simulink library "lib_accessory2"  (Simulink 4.1.1)
values from neighbouring files (symbols this model uses):
  logFlag = 1    [advSACompMaskInit.m]    (also in advSACompMaskInitR13.m)
undefined symbols (not defined in the file or in its folder): acc_abc_dutycycle, acc_abc_init, acc_ac_dutycycle, acc_ac_init, acc_acdc_inverter_eff, acc_alt_init, acc_dcdc_eff, acc_ef_dutycycle, acc_ef_init, acc_elec_eff, acc_elec_efficiency, acc_elec_pwr, acc_mech_eff, acc_mech_pwr, acc_mech_trq, acc_op_dutycycle, acc_op_init, acc_ps_dutycycle, acc_ps_init, acc_sindafile, acc_wp_dutycycle, acc_wp_init, amb_tmp, ess_on, fc_on, generalName, map_spd, max_pwr, tc_gc_to_fc_ratio, time_step, vc_idle_bool, vc_idle_spd, vinf
libraries: lib_cosimulation x29, lib_accessory2 x15, lib_outputs x11, simulink3 x10, lib_accessory x8, lib_etc x2
(part 4 of 5)

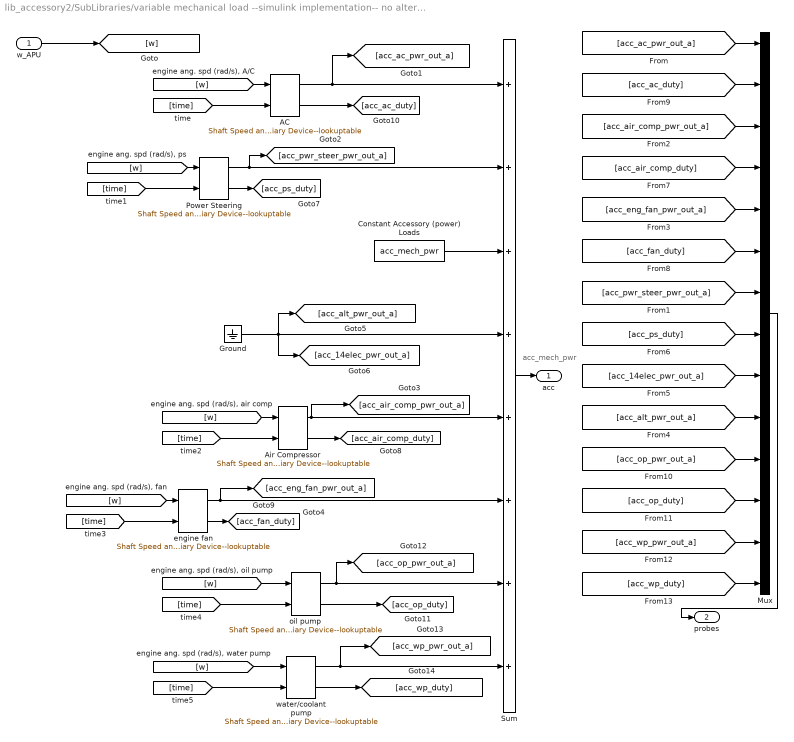
== system lib_accessory2/SubLibraries/variable mechanical load --simulink implementation-- no alternator ==
  note: acc_mech_pwr
  w_APU : Inport  Port=1  LatchInput=off
  AC : lib_accessory/SubLibraries/Shaft Speed and Time Loaded Auxiliary Device--lookuptable  fname=acc_ac_init  acc_duty=acc_ac_dutycycle
  Air Compressor : lib_accessory/SubLibraries/Shaft Speed and Time Loaded Auxiliary Device--lookuptable  fname=acc_abc_init  acc_duty=acc_abc_dutycycle
  Constant Accessory (power) Loads : Constant  Value=acc_mech_pwr
  Ground : Ground
  Mux : Mux  Inputs=14
  Power Steering : lib_accessory/SubLibraries/Shaft Speed and Time Loaded Auxiliary Device--lookuptable  fname=acc_ps_init  acc_duty=acc_ps_dutycycle
  Sum : Sum  Inputs=++++++++  SaturateOnIntegerOverflow=on
  engine fan : lib_accessory/SubLibraries/Shaft Speed and Time Loaded Auxiliary Device--lookuptable  fname=acc_ef_init  acc_duty=acc_ef_dutycycle
  oil pump : lib_accessory/SubLibraries/Shaft Speed and Time Loaded Auxiliary Device--lookuptable  fname=acc_op_init  acc_duty=acc_op_dutycycle
  water/coolant pump : lib_accessory/SubLibraries/Shaft Speed and Time Loaded Auxiliary Device--lookuptable  fname=acc_wp_init  acc_duty=acc_wp_dutycycle
  acc : Outport  Port=1
  probes : Outport  Port=2
  wires:
  [time] -> AC/2
  [w] -> AC/1
  AC/2 -> [acc_ac_duty]
  AC/1 -> Sum/1, [acc_ac_pwr_out_a]
  Constant Accessory (power) Loads/1 -> Sum/3
  Sum/1 -> acc/1
  Air Compressor/2 -> [acc_air_comp_duty]
  Air Compressor/1 -> Sum/5, [acc_air_comp_pwr_out_a]
  [w] -> Air Compressor/1
  [time] -> Air Compressor/2
  oil pump/1 -> [acc_op_pwr_out_a], Sum/7
  oil pump/2 -> [acc_op_duty]
  [time] -> oil pump/2
  [w] -> oil pump/1
  engine fan/2 -> [acc_fan_duty]
  [time] -> engine fan/2
  engine fan/1 -> Sum/6, [acc_eng_fan_pwr_out_a]
  [w] -> engine fan/1
  Power Steering/2 -> [acc_ps_duty]
  [w] -> Power Steering/1
  [time] -> Power Steering/2
  Power Steering/1 -> Sum/2, [acc_pwr_steer_pwr_out_a]
  w_APU/1 -> [w]
  [acc_ac_pwr_out_a] -> Mux/1
  Ground/1 -> Sum/4, [acc_alt_pwr_out_a], [acc_14elec_pwr_out_a]
  Mux/1 -> probes/1
  water/coolant pump/1 -> Sum/8, [acc_wp_pwr_out_a]
  [time] -> water/coolant pump/2
  [w] -> water/coolant pump/1
  water/coolant pump/2 -> [acc_wp_duty]
  [acc_ac_duty] -> Mux/2
  [acc_air_comp_pwr_out_a] -> Mux/3
  [acc_air_comp_duty] -> Mux/4
  [acc_eng_fan_pwr_out_a] -> Mux/5
  [acc_fan_duty] -> Mux/6
  [acc_pwr_steer_pwr_out_a] -> Mux/7
  [acc_ps_duty] -> Mux/8
  [acc_14elec_pwr_out_a] -> Mux/9
  [acc_alt_pwr_out_a] -> Mux/10
  [acc_op_pwr_out_a] -> Mux/11
  [acc_op_duty] -> Mux/12
  [acc_wp_pwr_out_a] -> Mux/13
  [acc_wp_duty] -> Mux/14

== system lib_accessory2/ACC ELEC <acce>/ACC ELEC model and interface/electrical accessory model ==
  note: Backward-Forward Models
  "requested electrical Power, out to the driveline (W)" : Inport  Port=1  LatchInput=off
  achieved power in from power source (W) : Inport  Port=2  LatchInput=off
  Block NOTES : Subsystem
      settings: RTWFcnNameOpts=Auto  RTWFileNameOpts=Auto
      mask Display: disp('Block\nNOTES')
  backward model : Subsystem
      settings: RTWFcnNameOpts=Auto  RTWFileNameOpts=Auto
  electrical power logging : lib_accessory2/SubLibraries/electrical power logging  eff=acc_mech_eff
      link override enhancedToWorkspace1/To Workspace: VariableName=acce_elec_pwr_in_a  SampleTime=-1  SaveFormat=Array
  enhancedToWorkspace : Subsystem  TreatAsAtomicUnit=on  mask(enhancedToWorkspace){generalName=generalName, specificName=elec_pwr_a, logFlag=logFlag}
      mask prompts: generalName "General Name [char-evaluated]"; specificName "Specific Name [char-literal]"; logFlag "Enable flag (1=on,0=off)"
      mask help: A wrapper for the Simulink "To Workspace" block that allows you to evaluate the name of the variable to log to workspace. This is useful to avoid the double logging errors that occur when you pull in two library models that attempt to log to the same variable.
      mask init:
      | enhancedToWsMaker
      settings: CopyFcn=breakLinkCopyFcn  ParentCloseFcn=breakLinkParCloseFcn  RTWFcnNameOpts=Auto  RTWFileNameOpts=Auto
      mask Help:
      | <h2>Enhanced To Workspace Block</h2>
      | <h3>Parameters</h3>
      | <UL>
      | <li><b>General Name:</b> This is the more general name of the variable. Variables are saved to the workspace as <i>generalName_specificName</i>. Note that this is an evaluated variable. If you would like to type in the value directly, it must be surrounded with single quotes. Otherwise you can input the name of a variable containing a char string.</li>
      | <li><b>Specific Name:</b> This is the specific name of the variable. Note that this is input as a char literal (i.e., you don't need quotes).</li>
      | <li><b>Enable Flag:</b> This flag should have the value of 0 or 1. If 0, the variable will not be logged to the workspace. If 1, the variable will be logged. This is done so that variable logging can be turned off to improve speed.</li>
      | </ul>
      | <h3>Overview</h3>
      | <p>The enhanced to workspace block was put together to allow one to dynamically resolve variable names at run time in simulink. This is most powerful when used in conjunction with a masked subsystem to allow multiple instances of that masked subsytem to be used in the same model. The strategy is to set the generalName in the block mask which will allow the block to change the general name for all variable logging on the fly.
      | <h3>Helper Files</h3>
      | <p>Three m-files are required by the enhancedToWorkspace block. These files are located in the &lt; ADVISOR root &gt;/GUI directory :
      | <ul>
      | <li><i>enhancedToWsMaker.m</i> This file runs the mask initialization for the block</li>
      | <li><i>breakLinkCopyFcn.m</i> This file is used by the block callback when the simulink block is copied. It is necessary to break the link to the enhancedToWorkspace similar to the To Workspace block in order for it to be able to configure itself. (Try copying simulink's To Workspace block--it is impossible to make a link)</li>
      | <li><i>breakLinkParCloseFcn.m</i> This file is similar to the breakLinkCopyFcn and is used when a parent system is closed</li>
      | </ul>
      | <hr>
      | 
      | <p>Created 2003-Jan-21, Michael Patrick O'Keefe, NREL</p>
      | 
      | <!--
      | <VARDEF>
      | <H3>var_name</H3>
      | <UL>
      | <LI><B>data type</B> data type here</LI>
      | <LI><B>units</B> units here</LI>
      | <LI><B>vehicle type</B> vehicle type here</LI>
      | <LI><B>description</B> description here</LI>
      | </UL>
      | </VARDEF>
      | -->
      mask Display: disp([generalName,'_',specificName])
  enhancedToWorkspace1 : Subsystem  TreatAsAtomicUnit=on  mask(enhancedToWorkspace){generalName=generalName, specificName=elec_pwr_r, logFlag=logFlag}
      mask prompts: generalName "General Name [char-evaluated]"; specificName "Specific Name [char-literal]"; logFlag "Enable flag (1=on,0=off)"
      mask help: A wrapper for the Simulink "To Workspace" block that allows you to evaluate the name of the variable to log to workspace. This is useful to avoid the double logging errors that occur when you pull in two library models that attempt to log to the same variable.
      mask init:
      | enhancedToWsMaker
      settings: CopyFcn=breakLinkCopyFcn  ParentCloseFcn=breakLinkParCloseFcn  RTWFcnNameOpts=Auto  RTWFileNameOpts=Auto
      mask Help:
      | <h2>Enhanced To Workspace Block</h2>
      | <h3>Parameters</h3>
      | <UL>
      | <li><b>General Name:</b> This is the more general name of the variable. Variables are saved to the workspace as <i>generalName_specificName</i>. Note that this is an evaluated variable. If you would like to type in the value directly, it must be surrounded with single quotes. Otherwise you can input the name of a variable containing a char string.</li>
      | <li><b>Specific Name:</b> This is the specific name of the variable. Note that this is input as a char literal (i.e., you don't need quotes).</li>
      | <li><b>Enable Flag:</b> This flag should have the value of 0 or 1. If 0, the variable will not be logged to the workspace. If 1, the variable will be logged. This is done so that variable logging can be turned off to improve speed.</li>
      | </ul>
      | <h3>Overview</h3>
      | <p>The enhanced to workspace block was put together to allow one to dynamically resolve variable names at run time in simulink. This is most powerful when used in conjunction with a masked subsystem to allow multiple instances of that masked subsytem to be used in the same model. The strategy is to set the generalName in the block mask which will allow the block to change the general name for all variable logging on the fly.
      | <h3>Helper Files</h3>
      | <p>Three m-files are required by the enhancedToWorkspace block. These files are located in the &lt; ADVISOR root &gt;/GUI directory :
      | <ul>
      | <li><i>enhancedToWsMaker.m</i> This file runs the mask initialization for the block</li>
      | <li><i>breakLinkCopyFcn.m</i> This file is used by the block callback when the simulink block is copied. It is necessary to break the link to the enhancedToWorkspace similar to the To Workspace block in order for it to be able to configure itself. (Try copying simulink's To Workspace block--it is impossible to make a link)</li>
      | <li><i>breakLinkParCloseFcn.m</i> This file is similar to the breakLinkCopyFcn and is used when a parent system is closed</li>
      | </ul>
      | <hr>
      | 
      | <p>Created 2003-Jan-21, Michael Patrick O'Keefe, NREL</p>
      | 
      | <!--
      | <VARDEF>
      | <H3>var_name</H3>
      | <UL>
      | <LI><B>data type</B> data type here</LI>
      | <LI><B>units</B> units here</LI>
      | <LI><B>vehicle type</B> vehicle type here</LI>
      | <LI><B>description</B> description here</LI>
      | </UL>
      | </VARDEF>
      | -->
      mask Display: disp([generalName,'_',specificName])
  forward model : Subsystem
      settings: RTWFcnNameOpts=Auto  RTWFileNameOpts=Auto
  "requested electrical Power, in from the power source (W)" : Outport  Port=1
  "achieved electrical Power, out to the driveline (W)" : Outport  Port=2
  tag scope: acc_elec_pwr_a=scoped, acc_elec_pwr_r=scoped
  wires:
  "requested electrical Power, out to the driveline (W)"/1 -> backward model/1(pwr_in)
  backward model/1(elec_out) -> "requested electrical Power, in from the power source (W)"/1
  achieved power in from power source (W)/1 -> forward model/1(pwr_in)
  forward model/1(pwr_out) -> "achieved electrical Power, out to the driveline (W)"/1
  backward model/2(elec_acc_out) -> [acc_elec_pwr_r], forward model/2(acc_pwr_in), enhancedToWorkspace1/1(In1)
  forward model/2(acc_pwr_out) -> [acc_elec_pwr_a], enhancedToWorkspace/1(In1), electrical power logging/1

== system lib_accessory2/ACC ELEC <acce>/ACC ELEC model and interface/signal annotator ==
  In1 : Inport  Port=1  LatchInput=off
  Out1 : Outport  Port=1
  wires:
  In1/1 -> Out1/1  "driveline_elec_pwr_r"

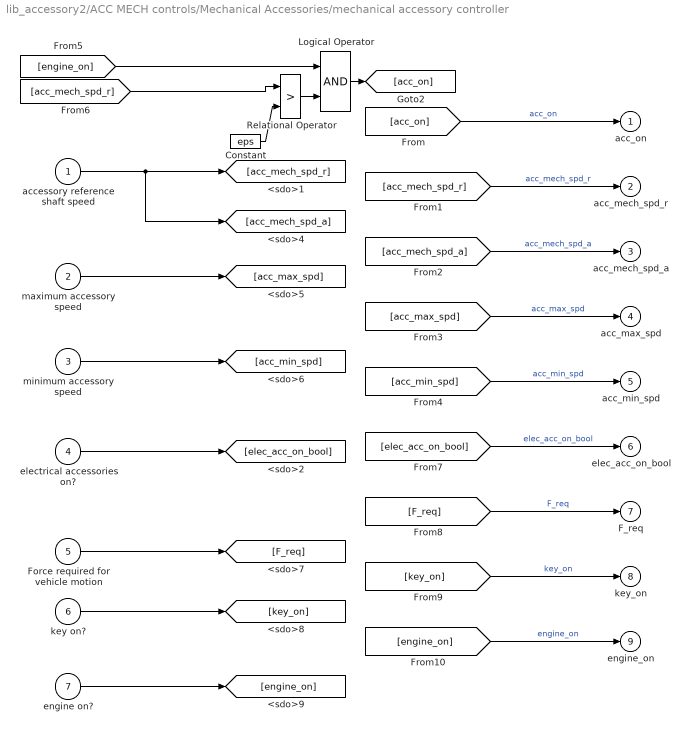
== system lib_accessory2/ACC MECH controls/Mechanical Accessories/mechanical accessory controller ==
  accessory reference shaft speed : Inport  Port=1  LatchInput=off
  maximum accessory speed : Inport  Port=2  LatchInput=off
  minimum accessory speed : Inport  Port=3  LatchInput=off
  electrical accessories on? : Inport  Port=4  LatchInput=off
  Force required for vehicle motion : Inport  Port=5  LatchInput=off
  key on? : Inport  Port=6  LatchInput=off
  engine on? : Inport  Port=7  LatchInput=off
  Constant : Constant  Value=eps
  Logical Operator : Logic  Operator=AND  Inputs=2
  Relational Operator : RelationalOperator  Operator=>
  acc_on : Outport  Port=1  InitialOutput=0
  acc_mech_spd_r : Outport  Port=2  InitialOutput=0
  acc_mech_spd_a : Outport  Port=3  InitialOutput=0
  acc_max_spd : Outport  Port=4  InitialOutput=0
  acc_min_spd : Outport  Port=5  InitialOutput=0
  elec_acc_on_bool : Outport  Port=6  InitialOutput=0
  F_req : Outport  Port=7  InitialOutput=0
  key_on : Outport  Port=8  InitialOutput=0
  engine_on : Outport  Port=9  InitialOutput=0
  wires:
  accessory reference shaft speed/1 -> [acc_mech_spd_r], [acc_mech_spd_a]
  maximum accessory speed/1 -> [acc_max_spd]
  minimum accessory speed/1 -> [acc_min_spd]
  electrical accessories on?/1 -> [elec_acc_on_bool]
  Force required for vehicle motion/1 -> [F_req]
  key on?/1 -> [key_on]
  engine on?/1 -> [engine_on]
  [acc_mech_spd_r] -> Relational Operator/1
  Constant/1 -> Relational Operator/2
  [engine_on] -> Logical Operator/1
  Relational Operator/1 -> Logical Operator/2
  Logical Operator/1 -> [acc_on]
  [acc_on] -> acc_on/1  "acc_on"
  [engine_on] -> engine_on/1  "engine_on"
  [key_on] -> key_on/1  "key_on"
  [F_req] -> F_req/1  "F_req"
  [elec_acc_on_bool] -> elec_acc_on_bool/1  "elec_acc_on_bool"
  [acc_min_spd] -> acc_min_spd/1  "acc_min_spd"
  [acc_max_spd] -> acc_max_spd/1  "acc_max_spd"
  [acc_mech_spd_a] -> acc_mech_spd_a/1  "acc_mech_spd_a"
  [acc_mech_spd_r] -> acc_mech_spd_r/1  "acc_mech_spd_r"

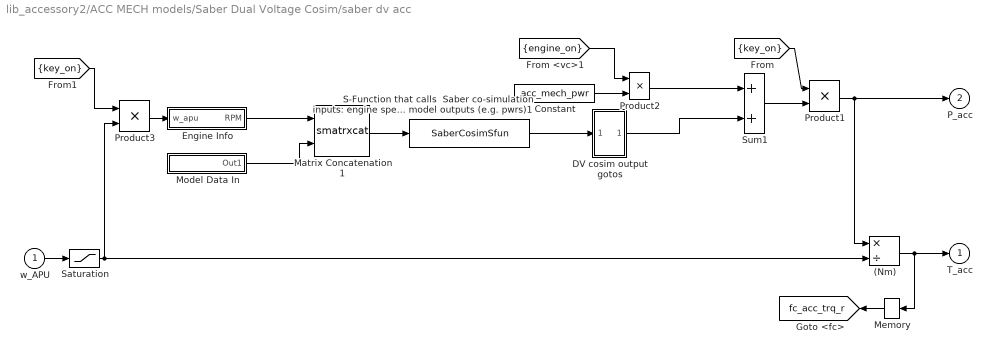
== system lib_accessory2/ACC MECH models/Saber Dual Voltage Cosim/saber dv acc ==
  w_APU : Inport  Port=1  LatchInput=off
  (Nm) : Product  Inputs=*/  Multiplication=Element-wise(.*)  SaturateOnIntegerOverflow=on
  Constant : Constant  Value=acc_mech_pwr
  DV cosim output gotos : Subsystem
      settings: RTWFcnNameOpts=Auto  RTWFileNameOpts=Auto
  Engine Info : Subsystem
      settings: RTWFcnNameOpts=Auto  RTWFileNameOpts=Auto
  Matrix Concatenation1 : S-Function  FunctionName=smatrxcat  Parameters=numInports,catMethod  PortCounts=[]  SFunctionModules=''  mask(Matrix Concatenation){numInports=2, catMethod=Horizontal}
      mask prompts: numInports "Number of inputs:"; catMethod "Concatenation method:"
      mask help: Perform horizontal or vertical concatenation. 1-D vector input signals are treated as column vectors, i.e., [Mx1] matrices. The output is always a matrix.
      mask init:
      | xy = matrxcatmask('icon');
      mask StyleString: edit,popup(Horizontal|Vertical)
      mask Display:
      | plot(xy.x,xy.y);
      | text(0.15,0.86,xy.label);
  Memory : Memory  Orientation=left  X0=0  InheritSampleTime=off
      settings: RTWStateStorageClass=Auto
  Model Data In : Subsystem
      settings: RTWFcnNameOpts=Auto  RTWFileNameOpts=Auto
      mask Display: disp('14V/42V acc')
  Product1 : Product  Inputs=2  Multiplication=Element-wise(.*)  SaturateOnIntegerOverflow=on
  Product2 : Product  Inputs=2  Multiplication=Element-wise(.*)  SaturateOnIntegerOverflow=on
  Product3 : Product  Inputs=2  Multiplication=Element-wise(.*)  SaturateOnIntegerOverflow=on
  S-Function that calls  Saber co-simulation inputs: engine speed (rad/s) load parameters outputs: accessory power model outputs (e.g. pwrs)1 : S-Function  FunctionName=SaberCosimSfun  Parameters=vinf.tmppath,time_step,'SaberCosimIO_DV'  PortCounts=[]  SFunctionModules=''
  Saturation : Saturate  UpperLimit=inf  LowerLimit=0  LinearizeAsGain=on
  Sum1 : Sum  Inputs=++  SaturateOnIntegerOverflow=on
  T_acc : Outport  Port=1  InitialOutput=0
  P_acc : Outport  Port=2  InitialOutput=0
  tag scope: fc_acc_trq_r=global
  wires:
  Product3/1 -> Engine Info/1(w_apu)
  [key_on] -> Product3/1
  DV cosim output gotos/1(Out1) -> Sum1/2
  Product1/1 -> (Nm)/1, P_acc/1
  [key_on] -> Product1/1
  Sum1/1 -> Product1/2
  Product2/1 -> Sum1/1
  [engine_on] -> Product2/1
  Constant/1 -> Product2/2
  (Nm)/1 -> T_acc/1, Memory/1
  Memory/1 -> [fc_acc_trq_r]
  w_APU/1 -> Saturation/1
  Saturation/1 -> Product3/2, (Nm)/2
  S-Function that calls  Saber co-simulation inputs: engine speed (rad/s) load parameters outputs: accessory power model outputs (e.g. pwrs)1/1 -> DV cosim output gotos/1(In1)
  Matrix Concatenation1/1 -> S-Function that calls  Saber co-simulation inputs: engine speed (rad/s) load parameters outputs: accessory power model outputs (e.g. pwrs)1/1
  Engine Info/1(RPM) -> Matrix Concatenation1/1
  Model Data In/1(Out1) -> Matrix Concatenation1/2

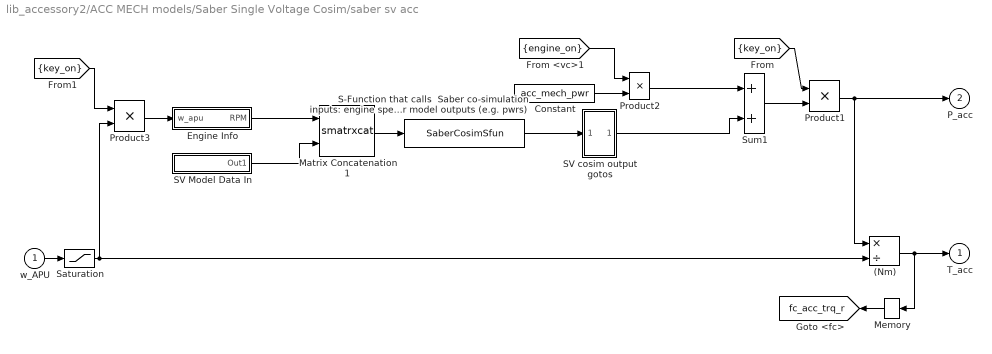
== system lib_accessory2/ACC MECH models/Saber Single Voltage Cosim/saber sv acc ==
  w_APU : Inport  Port=1  LatchInput=off
  (Nm) : Product  Inputs=*/  Multiplication=Element-wise(.*)  SaturateOnIntegerOverflow=on
  Constant : Constant  Value=acc_mech_pwr
  Engine Info : Subsystem
      settings: RTWFcnNameOpts=Auto  RTWFileNameOpts=Auto
  Matrix Concatenation1 : S-Function  FunctionName=smatrxcat  Parameters=numInports,catMethod  PortCounts=[]  SFunctionModules=''  mask(Matrix Concatenation){numInports=2, catMethod=Horizontal}
      mask prompts: numInports "Number of inputs:"; catMethod "Concatenation method:"
      mask help: Perform horizontal or vertical concatenation. 1-D vector input signals are treated as column vectors, i.e., [Mx1] matrices. The output is always a matrix.
      mask init:
      | xy = matrxcatmask('icon');
      mask StyleString: edit,popup(Horizontal|Vertical)
      mask Display:
      | plot(xy.x,xy.y);
      | text(0.15,0.86,xy.label);
  Memory : Memory  Orientation=left  X0=0  InheritSampleTime=off
      settings: RTWStateStorageClass=Auto
  Product1 : Product  Inputs=2  Multiplication=Element-wise(.*)  SaturateOnIntegerOverflow=on
  Product2 : Product  Inputs=2  Multiplication=Element-wise(.*)  SaturateOnIntegerOverflow=on
  Product3 : Product  Inputs=2  Multiplication=Element-wise(.*)  SaturateOnIntegerOverflow=on
  S-Function that calls  Saber co-simulation inputs: engine speed (rad/s) load parameters outputs: accessory power model outputs (e.g. pwrs) : S-Function  FunctionName=SaberCosimSfun  Parameters=vinf.tmppath,time_step,'SaberCosimIO_SV'  PortCounts=[]  SFunctionModules=''
  SV Model Data In : Subsystem
      settings: RTWFcnNameOpts=Auto  RTWFileNameOpts=Auto
      mask Display: disp('14V acc')
  SV cosim output gotos : Subsystem
      settings: RTWFcnNameOpts=Auto  RTWFileNameOpts=Auto
  Saturation : Saturate  UpperLimit=inf  LowerLimit=0  LinearizeAsGain=on
  Sum1 : Sum  Inputs=++  SaturateOnIntegerOverflow=on
  T_acc : Outport  Port=1  InitialOutput=0
  P_acc : Outport  Port=2  InitialOutput=0
  tag scope: fc_acc_trq_r=global
  wires:
  Product3/1 -> Engine Info/1(w_apu)
  [key_on] -> Product3/1
  SV cosim output gotos/1(Out1) -> Sum1/2
  SV Model Data In/1(Out1) -> Matrix Concatenation1/2
  Engine Info/1(RPM) -> Matrix Concatenation1/1
  Matrix Concatenation1/1 -> S-Function that calls  Saber co-simulation inputs: engine speed (rad/s) load parameters outputs: accessory power model outputs (e.g. pwrs)/1
  S-Function that calls  Saber co-simulation inputs: engine speed (rad/s) load parameters outputs: accessory power model outputs (e.g. pwrs)/1 -> SV cosim output gotos/1(In1)
  Saturation/1 -> Product3/2, (Nm)/2
  w_APU/1 -> Saturation/1
  Memory/1 -> [fc_acc_trq_r]
  (Nm)/1 -> Memory/1, T_acc/1
  Constant/1 -> Product2/2
  [engine_on] -> Product2/1
  Product2/1 -> Sum1/1
  Sum1/1 -> Product1/2
  [key_on] -> Product1/1
  Product1/1 -> P_acc/1, (Nm)/1

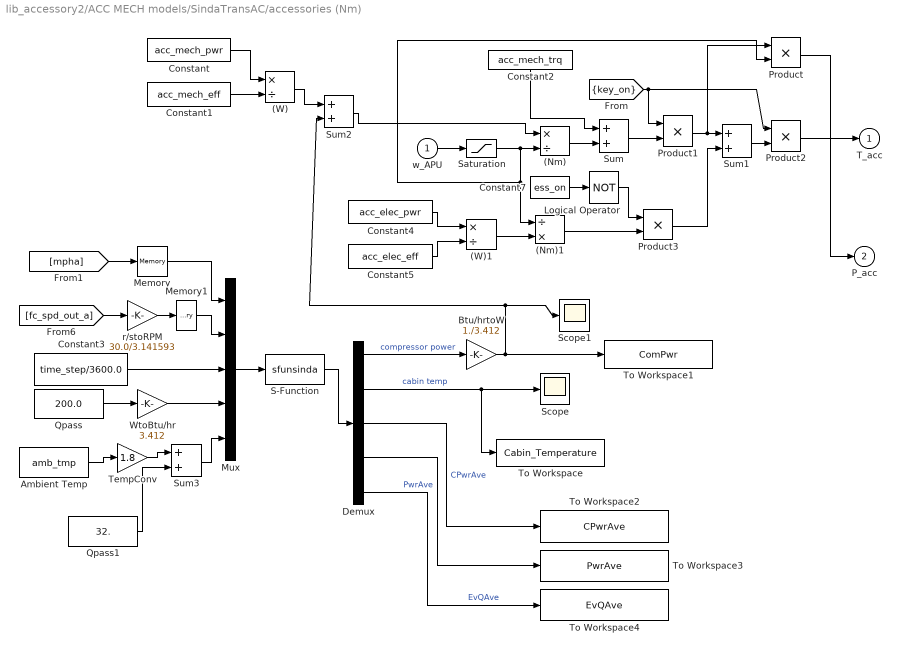
== system lib_accessory2/ACC MECH models/SindaTransAC/accessories (Nm) ==
  w_APU : Inport  Port=1  LatchInput=off
  (Nm) : Product  Inputs=*/  Multiplication=Element-wise(.*)  SaturateOnIntegerOverflow=on
  (Nm)1 : Product  Inputs=/*  Multiplication=Element-wise(.*)  SaturateOnIntegerOverflow=on
  (W) : Product  Inputs=*/  Multiplication=Element-wise(.*)  SaturateOnIntegerOverflow=on
  (W)1 : Product  Inputs=*/  Multiplication=Element-wise(.*)  SaturateOnIntegerOverflow=on
  Ambient Temp : Constant  Value=amb_tmp
  Btu/hrtoW : Gain  Gain=1./3.412  Multiplication=Element-wise(K.*u)  SaturateOnIntegerOverflow=on
  Constant : Constant  Value=acc_mech_pwr
  Constant1 : Constant  Value=acc_mech_eff
  Constant2 : Constant  Orientation=down  Value=acc_mech_trq
  Constant3 : Constant  Value=time_step/3600.0
  Constant4 : Constant  Value=acc_elec_pwr
  Constant5 : Constant  Value=acc_elec_eff
  Constant7 : Constant  Value=ess_on
  Demux : Demux  Outputs=5  BusSelectionMode=off
  Logical Operator : Logic  Operator=NOT  Inputs=2
  Memory : Memory  X0=45.0  InheritSampleTime=off
      settings: RTWStateStorageClass=Auto
  Memory1 : Memory  X0=600.  InheritSampleTime=off
      settings: RTWStateStorageClass=Auto
  Mux : Mux  Inputs=5
  Product{,1..3} (4 alike) : Product  Inputs=2  Multiplication=Element-wise(.*)  SaturateOnIntegerOverflow=on
  Qpass : Constant  Value=200.0
  Qpass1 : Constant  Value=32.
  S-Function : S-Function  FunctionName=sfunsinda  Parameters=sindafile  PortCounts=[]  SFunctionModules=''
  Saturation : Saturate  UpperLimit=inf  LowerLimit=vc_idle_spd+eps  LinearizeAsGain=on
  Scope : Scope
      settings: TimeRange=auto  YMin=130  YMax=170  SaveToWorkspace=off  SaveName=ScopeData  LimitDataPoints=on  MaxDataPoints=5000
  Scope1 : Scope
      settings: TimeRange=auto  YMin=-5  YMax=5  SaveToWorkspace=off  SaveName=ScopeData  LimitDataPoints=on  MaxDataPoints=5000
  Sum{,1..3} (4 alike) : Sum  Inputs=++  SaturateOnIntegerOverflow=on
  TempConv : Gain  Gain=1.8  Multiplication=Element-wise(K.*u)  SaturateOnIntegerOverflow=on
  To Workspace : ToWorkspace  VariableName=Cabin_Temperature  SampleTime=-1  SaveFormat=Array
  To Workspace1 : ToWorkspace  VariableName=ComPwr  SampleTime=-1  SaveFormat=Array
  To Workspace2 : ToWorkspace  VariableName=CPwrAve  SampleTime=-1  SaveFormat=Array
  To Workspace3 : ToWorkspace  VariableName=PwrAve  SampleTime=-1  SaveFormat=Array
  To Workspace4 : ToWorkspace  VariableName=EvQAve  SampleTime=-1  SaveFormat=Array
  WtoBtu/hr : Gain  Gain=3.412  Multiplication=Element-wise(K.*u)  SaturateOnIntegerOverflow=on
  r/stoRPM : Gain  Gain=30.0/3.141593  Multiplication=Element-wise(K.*u)  SaturateOnIntegerOverflow=on
  T_acc : Outport  Port=1  InitialOutput=0
  P_acc : Outport  Port=2  InitialOutput=0
  wires:
  Mux/1 -> S-Function/1
  S-Function/1 -> Demux/1
  [fc_spd_out_a] -> r/stoRPM/1
  Qpass/1 -> WtoBtu/hr/1
  WtoBtu/hr/1 -> Mux/4
  Product1/1 -> Product/1, Sum1/1
  Sum1/1 -> Product2/2
  Logical Operator/1 -> Product3/1
  Product3/1 -> Sum1/2
  Product/1 -> P_acc/1
  (Nm)1/1 -> Product3/2
  Constant7/1 -> Logical Operator/1
  (W)1/1 -> (Nm)1/2
  Constant4/1 -> (W)1/1
  Constant5/1 -> (W)1/2
  Product2/1 -> T_acc/1
  [key_on] -> Product2/1, Product1/1
  Sum/1 -> Product1/2
  (Nm)/1 -> Sum/2
  Saturation/1 -> Product/2, (Nm)1/1, (Nm)/2
  w_APU/1 -> Saturation/1
  Constant2/1 -> Sum/1
  (W)/1 -> Sum2/1
  Sum2/1 -> (Nm)/1
  Constant/1 -> (W)/1
  Constant1/1 -> (W)/2
  Demux/2 -> To Workspace/1, Scope/1  "cabin temp"
  Ambient Temp/1 -> TempConv/1
  TempConv/1 -> Sum3/1
  Qpass1/1 -> Sum3/2
  Sum3/1 -> Mux/5
  Demux/1 -> Btu/hrtoW/1  "compressor power"
  [mpha] -> Memory/1
  Memory/1 -> Mux/1
  r/stoRPM/1 -> Memory1/1
  Memory1/1 -> Mux/2
  Constant3/1 -> Mux/3
  Btu/hrtoW/1 -> Sum2/2, Scope1/1, To Workspace1/1
  Demux/3 -> To Workspace2/1  "CPwrAve"
  Demux/4 -> To Workspace3/1  "PwrAve"
  Demux/5 -> To Workspace4/1  "EvQAve"

== system lib_accessory2/ACC MECH <accm>/mechanical accessory model and interface/Block NOTES ==

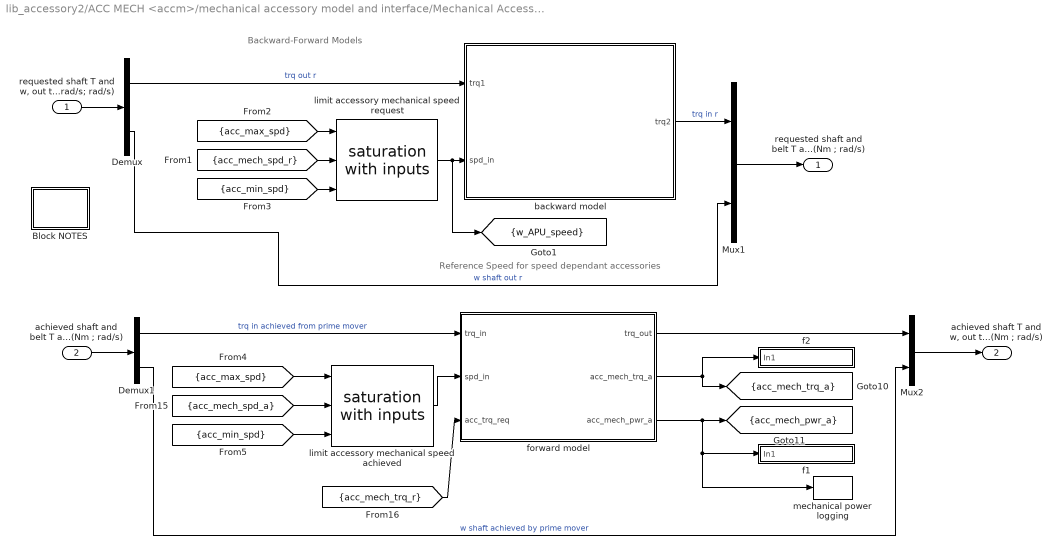
== system lib_accessory2/ACC MECH <accm>/mechanical accessory model and interface/Mechanical Accessory model ==
  note: Backward-Forward Models
  note: Reference Speed for speed dependant accessories
  "requested shaft T and w, out to the driveline  (Nm ; rad/s; rad/s)" : Inport  Port=1  LatchInput=off
  "achieved shaft and belt T and w, in from the prime mover (Nm ; rad/s)" : Inport  Port=2  LatchInput=off
  Block NOTES : Subsystem
      settings: RTWFcnNameOpts=Auto  RTWFileNameOpts=Auto
      mask Display: disp('Block\nNOTES')
  Demux : Demux  Outputs=2  BusSelectionMode=off
  Demux1 : Demux  Outputs=2  BusSelectionMode=off
  Mux1 : Mux  Inputs=2
  Mux2 : Mux  Inputs=2
  backward model : Subsystem
      settings: RTWFcnNameOpts=Auto  RTWFileNameOpts=Auto
  f1 : Subsystem  TreatAsAtomicUnit=on  mask(enhancedToWorkspace){generalName=generalName, specificName=mech_pwr_a, logFlag=logFlag}
      mask prompts: generalName "General Name [char-evaluated]"; specificName "Specific Name [char-literal]"; logFlag "Enable flag (1=on,0=off)"
      mask help: A wrapper for the Simulink "To Workspace" block that allows you to evaluate the name of the variable to log to workspace. This is useful to avoid the double logging errors that occur when you pull in two library models that attempt to log to the same variable.
      mask init:
      | enhancedToWsMaker
      settings: CopyFcn=breakLinkCopyFcn  ParentCloseFcn=breakLinkParCloseFcn  RTWFcnNameOpts=Auto  RTWFileNameOpts=Auto
      mask Help:
      | <h2>Enhanced To Workspace Block</h2>
      | <h3>Parameters</h3>
      | <UL>
      | <li><b>General Name:</b> This is the more general name of the variable. Variables are saved to the workspace as <i>generalName_specificName</i>. Note that this is an evaluated variable. If you would like to type in the value directly, it must be surrounded with single quotes. Otherwise you can input the name of a variable containing a char string.</li>
      | <li><b>Specific Name:</b> This is the specific name of the variable. Note that this is input as a char literal (i.e., you don't need quotes).</li>
      | <li><b>Enable Flag:</b> This flag should have the value of 0 or 1. If 0, the variable will not be logged to the workspace. If 1, the variable will be logged. This is done so that variable logging can be turned off to improve speed.</li>
      | </ul>
      | <h3>Overview</h3>
      | <p>The enhanced to workspace block was put together to allow one to dynamically resolve variable names at run time in simulink. This is most powerful when used in conjunction with a masked subsystem to allow multiple instances of that masked subsytem to be used in the same model. The strategy is to set the generalName in the block mask which will allow the block to change the general name for all variable logging on the fly.
      | <h3>Helper Files</h3>
      | <p>Three m-files are required by the enhancedToWorkspace block. These files are located in the &lt; ADVISOR root &gt;/GUI directory :
      | <ul>
      | <li><i>enhancedToWsMaker.m</i> This file runs the mask initialization for the block</li>
      | <li><i>breakLinkCopyFcn.m</i> This file is used by the block callback when the simulink block is copied. It is necessary to break the link to the enhancedToWorkspace similar to the To Workspace block in order for it to be able to configure itself. (Try copying simulink's To Workspace block--it is impossible to make a link)</li>
      | <li><i>breakLinkParCloseFcn.m</i> This file is similar to the breakLinkCopyFcn and is used when a parent system is closed</li>
      | </ul>
      | <hr>
      | 
      | <p>Created 2003-Jan-21, Michael Patrick O'Keefe, NREL</p>
      | 
      | <!--
      | <VARDEF>
      | <H3>var_name</H3>
      | <UL>
      | <LI><B>data type</B> data type here</LI>
      | <LI><B>units</B> units here</LI>
      | <LI><B>vehicle type</B> vehicle type here</LI>
      | <LI><B>description</B> description here</LI>
      | </UL>
      | </VARDEF>
      | -->
      mask Display: disp([generalName,'_',specificName])
  f2 : Subsystem  TreatAsAtomicUnit=on  mask(enhancedToWorkspace){generalName=generalName, specificName=mech_trq_a, logFlag=logFlag}
      mask prompts: generalName "General Name [char-evaluated]"; specificName "Specific Name [char-literal]"; logFlag "Enable flag (1=on,0=off)"
      mask help: A wrapper for the Simulink "To Workspace" block that allows you to evaluate the name of the variable to log to workspace. This is useful to avoid the double logging errors that occur when you pull in two library models that attempt to log to the same variable.
      mask init:
      | enhancedToWsMaker
      settings: CopyFcn=breakLinkCopyFcn  ParentCloseFcn=breakLinkParCloseFcn  RTWFcnNameOpts=Auto  RTWFileNameOpts=Auto
      mask Help:
      | <h2>Enhanced To Workspace Block</h2>
      | <h3>Parameters</h3>
      | <UL>
      | <li><b>General Name:</b> This is the more general name of the variable. Variables are saved to the workspace as <i>generalName_specificName</i>. Note that this is an evaluated variable. If you would like to type in the value directly, it must be surrounded with single quotes. Otherwise you can input the name of a variable containing a char string.</li>
      | <li><b>Specific Name:</b> This is the specific name of the variable. Note that this is input as a char literal (i.e., you don't need quotes).</li>
      | <li><b>Enable Flag:</b> This flag should have the value of 0 or 1. If 0, the variable will not be logged to the workspace. If 1, the variable will be logged. This is done so that variable logging can be turned off to improve speed.</li>
      | </ul>
      | <h3>Overview</h3>
      | <p>The enhanced to workspace block was put together to allow one to dynamically resolve variable names at run time in simulink. This is most powerful when used in conjunction with a masked subsystem to allow multiple instances of that masked subsytem to be used in the same model. The strategy is to set the generalName in the block mask which will allow the block to change the general name for all variable logging on the fly.
      | <h3>Helper Files</h3>
      | <p>Three m-files are required by the enhancedToWorkspace block. These files are located in the &lt; ADVISOR root &gt;/GUI directory :
      | <ul>
      | <li><i>enhancedToWsMaker.m</i> This file runs the mask initialization for the block</li>
      | <li><i>breakLinkCopyFcn.m</i> This file is used by the block callback when the simulink block is copied. It is necessary to break the link to the enhancedToWorkspace similar to the To Workspace block in order for it to be able to configure itself. (Try copying simulink's To Workspace block--it is impossible to make a link)</li>
      | <li><i>breakLinkParCloseFcn.m</i> This file is similar to the breakLinkCopyFcn and is used when a parent system is closed</li>
      | </ul>
      | <hr>
      | 
      | <p>Created 2003-Jan-21, Michael Patrick O'Keefe, NREL</p>
      | 
      | <!--
      | <VARDEF>
      | <H3>var_name</H3>
      | <UL>
      | <LI><B>data type</B> data type here</LI>
      | <LI><B>units</B> units here</LI>
      | <LI><B>vehicle type</B> vehicle type here</LI>
      | <LI><B>description</B> description here</LI>
      | </UL>
      | </VARDEF>
      | -->
      mask Display: disp([generalName,'_',specificName])
  forward model : Subsystem
      settings: RTWFcnNameOpts=Auto  RTWFileNameOpts=Auto
  limit accessory mechanical speed achieved : lib_etc/saturation with inputs
      settings: RTWFcnNameOpts=Auto  RTWFileNameOpts=Auto
  limit accessory mechanical speed request : lib_etc/saturation with inputs
      settings: RTWFcnNameOpts=Auto  RTWFileNameOpts=Auto
  mechanical power logging : lib_accessory2/SubLibraries/mechanical power logging  eff=acc_mech_eff
  "requested shaft and belt T and w, in from the prime mover (Nm ; rad/s)" : Outport  Port=1
  "achieved shaft T and w, out to the driveline (Nm ; rad/s)" : Outport  Port=2
  tag scope: acc_mech_pwr_a=scoped, acc_mech_trq_a=scoped, w_APU_speed=scoped
  wires:
  Demux1/2 -> Mux2/2  "w shaft achieved by prime mover"
  Demux1/1 -> forward model/1(trq_in)  "trq in achieved from prime mover"
  forward model/1(trq_out) -> Mux2/1
  backward model/1(trq2) -> Mux1/1  "trq in r"
  Demux/2 -> Mux1/2  "w shaft out r"
  Demux/1 -> backward model/1(trq1)  "trq out r"
  "requested shaft T and w, out to the driveline  (Nm ; rad/s; rad/s)"/1 -> Demux/1
  "achieved shaft and belt T and w, in from the prime mover (Nm ; rad/s)"/1 -> Demux1/1
  Mux1/1 -> "requested shaft and belt T and w, in from the prime mover (Nm ; rad/s)"/1
  Mux2/1 -> "achieved shaft T and w, out to the driveline (Nm ; rad/s)"/1
  forward model/2(acc_mech_trq_a) -> [acc_mech_trq_a], f2/1(In1)
  forward model/3(acc_mech_pwr_a) -> [acc_mech_pwr_a], f1/1(In1), mechanical power logging/1
  [acc_mech_trq_r] -> forward model/3(acc_trq_req)
  [acc_mech_spd_r] -> limit accessory mechanical speed request/2
  limit accessory mechanical speed request/1 -> backward model/2(spd_in), [w_APU_speed]
  [acc_max_spd] -> limit accessory mechanical speed request/1
  [acc_min_spd] -> limit accessory mechanical speed request/3
  limit accessory mechanical speed achieved/1 -> forward model/2(spd_in)
  [acc_mech_spd_a] -> limit accessory mechanical speed achieved/2
  [acc_max_spd] -> limit accessory mechanical speed achieved/1
  [acc_min_spd] -> limit accessory mechanical speed achieved/3

== system lib_accessory2/ACC MECH <accm>/mechanical accessory model and interface/help ==

== system lib_accessory2/ACC MECH <accm>/mechanical accessory model and interface/signal annotator ==
  In1 : Inport  Port=1  LatchInput=off
  Demux : Demux  Outputs=2  BusSelectionMode=off
  Mux : Mux  Inputs=2
  enhancedToWorkspace : Subsystem  TreatAsAtomicUnit=on  mask(enhancedToWorkspace){generalName=generalName, specificName=pre_acc_spd_out_r, logFlag=logFlag}
      mask prompts: generalName "General Name [char-evaluated]"; specificName "Specific Name [char-literal]"; logFlag "Enable flag (1=on,0=off)"
      mask help: A wrapper for the Simulink "To Workspace" block that allows you to evaluate the name of the variable to log to workspace. This is useful to avoid the double logging errors that occur when you pull in two library models that attempt to log to the same variable.
      mask init:
      | enhancedToWsMaker
      settings: CopyFcn=breakLinkCopyFcn  ParentCloseFcn=breakLinkParCloseFcn  RTWFcnNameOpts=Auto  RTWFileNameOpts=Auto
      mask Help:
      | <h2>Enhanced To Workspace Block</h2>
      | <h3>Parameters</h3>
      | <UL>
      | <li><b>General Name:</b> This is the more general name of the variable. Variables are saved to the workspace as <i>generalName_specificName</i>. Note that this is an evaluated variable. If you would like to type in the value directly, it must be surrounded with single quotes. Otherwise you can input the name of a variable containing a char string.</li>
      | <li><b>Specific Name:</b> This is the specific name of the variable. Note that this is input as a char literal (i.e., you don't need quotes).</li>
      | <li><b>Enable Flag:</b> This flag should have the value of 0 or 1. If 0, the variable will not be logged to the workspace. If 1, the variable will be logged. This is done so that variable logging can be turned off to improve speed.</li>
      | </ul>
      | <h3>Overview</h3>
      | <p>The enhanced to workspace block was put together to allow one to dynamically resolve variable names at run time in simulink. This is most powerful when used in conjunction with a masked subsystem to allow multiple instances of that masked subsytem to be used in the same model. The strategy is to set the generalName in the block mask which will allow the block to change the general name for all variable logging on the fly.
      | <h3>Helper Files</h3>
      | <p>Three m-files are required by the enhancedToWorkspace block. These files are located in the &lt; ADVISOR root &gt;/GUI directory :
      | <ul>
      | <li><i>enhancedToWsMaker.m</i> This file runs the mask initialization for the block</li>
      | <li><i>breakLinkCopyFcn.m</i> This file is used by the block callback when the simulink block is copied. It is necessary to break the link to the enhancedToWorkspace similar to the To Workspace block in order for it to be able to configure itself. (Try copying simulink's To Workspace block--it is impossible to make a link)</li>
      | <li><i>breakLinkParCloseFcn.m</i> This file is similar to the breakLinkCopyFcn and is used when a parent system is closed</li>
      | </ul>
      | <hr>
      | 
      | <p>Created 2003-Jan-21, Michael Patrick O'Keefe, NREL</p>
      | 
      | <!--
      | <VARDEF>
      | <H3>var_name</H3>
      | <UL>
      | <LI><B>data type</B> data type here</LI>
      | <LI><B>units</B> units here</LI>
      | <LI><B>vehicle type</B> vehicle type here</LI>
      | <LI><B>description</B> description here</LI>
      | </UL>
      | </VARDEF>
      | -->
      mask Display: disp([generalName,'_',specificName])
  enhancedToWorkspace1 : Subsystem  TreatAsAtomicUnit=on  mask(enhancedToWorkspace){generalName=generalName, specificName=pre_acc_trq_out_r, logFlag=logFlag}
      mask prompts: generalName "General Name [char-evaluated]"; specificName "Specific Name [char-literal]"; logFlag "Enable flag (1=on,0=off)"
      mask help: A wrapper for the Simulink "To Workspace" block that allows you to evaluate the name of the variable to log to workspace. This is useful to avoid the double logging errors that occur when you pull in two library models that attempt to log to the same variable.
      mask init:
      | enhancedToWsMaker
      settings: CopyFcn=breakLinkCopyFcn  ParentCloseFcn=breakLinkParCloseFcn  RTWFcnNameOpts=Auto  RTWFileNameOpts=Auto
      mask Help:
      | <h2>Enhanced To Workspace Block</h2>
      | <h3>Parameters</h3>
      | <UL>
      | <li><b>General Name:</b> This is the more general name of the variable. Variables are saved to the workspace as <i>generalName_specificName</i>. Note that this is an evaluated variable. If you would like to type in the value directly, it must be surrounded with single quotes. Otherwise you can input the name of a variable containing a char string.</li>
      | <li><b>Specific Name:</b> This is the specific name of the variable. Note that this is input as a char literal (i.e., you don't need quotes).</li>
      | <li><b>Enable Flag:</b> This flag should have the value of 0 or 1. If 0, the variable will not be logged to the workspace. If 1, the variable will be logged. This is done so that variable logging can be turned off to improve speed.</li>
      | </ul>
      | <h3>Overview</h3>
      | <p>The enhanced to workspace block was put together to allow one to dynamically resolve variable names at run time in simulink. This is most powerful when used in conjunction with a masked subsystem to allow multiple instances of that masked subsytem to be used in the same model. The strategy is to set the generalName in the block mask which will allow the block to change the general name for all variable logging on the fly.
      | <h3>Helper Files</h3>
      | <p>Three m-files are required by the enhancedToWorkspace block. These files are located in the &lt; ADVISOR root &gt;/GUI directory :
      | <ul>
      | <li><i>enhancedToWsMaker.m</i> This file runs the mask initialization for the block</li>
      | <li><i>breakLinkCopyFcn.m</i> This file is used by the block callback when the simulink block is copied. It is necessary to break the link to the enhancedToWorkspace similar to the To Workspace block in order for it to be able to configure itself. (Try copying simulink's To Workspace block--it is impossible to make a link)</li>
      | <li><i>breakLinkParCloseFcn.m</i> This file is similar to the breakLinkCopyFcn and is used when a parent system is closed</li>
      | </ul>
      | <hr>
      | 
      | <p>Created 2003-Jan-21, Michael Patrick O'Keefe, NREL</p>
      | 
      | <!--
      | <VARDEF>
      | <H3>var_name</H3>
      | <UL>
      | <LI><B>data type</B> data type here</LI>
      | <LI><B>units</B> units here</LI>
      | <LI><B>vehicle type</B> vehicle type here</LI>
      | <LI><B>description</B> description here</LI>
      | </UL>
      | </VARDEF>
      | -->
      mask Display: disp([generalName,'_',specificName])
  Out1 : Outport  Port=1
  wires:
  In1/1 -> Demux/1
  Demux/1 -> enhancedToWorkspace1/1(In1), Mux/1  "macc_trq_out_r"
  Demux/2 -> enhancedToWorkspace/1(In1), Mux/2  "macc_spd_out_r"
  Mux/1 -> Out1/1

== system lib_accessory2/Elec Aux Loads HiV Pwr/Starter/Starter ==
  14 V : Constant  Value=vinf.AuxLoads.Starter.HiV
  Hit  Crossing : HitCross  HitCrossingOffset=0  HitCrossingDirection=rising  ShowOutputPort=on
  Memory : Memory  X0=fc_on  InheritSampleTime=off
      settings: RTWStateStorageClass=Auto
  On : Constant  Value=vinf.AuxLoads.Starter.On
  Product1 : Product  Inputs=4  Multiplication=Element-wise(.*)  SaturateOnIntegerOverflow=on
  Subsystem : Subsystem
      settings: RTWFcnNameOpts=Auto  RTWFileNameOpts=Auto
  Starter_OnOff_Control : Outport  Port=1
  wires:
  14 V/1 -> Product1/2
  Subsystem/1(Out1) -> Product1/3
  Product1/1 -> Starter_OnOff_Control/1
  On/1 -> Product1/1
  [key_on] -> Product1/4
  [time] -> Subsystem/2(In2)
  [engine_on] -> Memory/1
  Hit  Crossing/1 -> Subsystem/1(In1)
  Memory/1 -> Hit  Crossing/1

== system lib_accessory2/SubLibraries/Shaft Speed and Time Loaded Auxiliary Device/device duty  schedule by time ==
  distance travelled (m) : Inport  Port=1  LatchInput=off
  Fcn1 : Fcn  Expr=rem(u[1],period)
  Look-Up Table : Lookup  InputValues=t  OutputValues=y
  out_1 : Outport  Port=1  InitialOutput=0
  wires:
  Look-Up Table/1 -> out_1/1
  Fcn1/1 -> Look-Up Table/1
  distance travelled (m)/1 -> Fcn1/1

== system lib_accessory2/SubLibraries/Shaft Speed and Time Loaded Auxiliary Device--lookuptable/device duty  schedule by time ==
  distance travelled (m) : Inport  Port=1  LatchInput=off
  Fcn1 : Fcn  Expr=rem(u[1],period)
  Look-Up Table : Lookup  InputValues=t  OutputValues=y
  out_1 : Outport  Port=1  InitialOutput=0
  wires:
  distance travelled (m)/1 -> Fcn1/1
  Fcn1/1 -> Look-Up Table/1
  Look-Up Table/1 -> out_1/1

== system lib_accessory2/SubLibraries/electrical power logging/enhancedToWorkspace ==
  In1 : Inport  Port=1  LatchInput=off
  Terminator : Terminator
  wires:
  In1/1 -> Terminator/1

== system lib_accessory2/SubLibraries/electrical power logging/enhancedToWorkspace1 ==
  In1 : Inport  Port=1  LatchInput=off
  Terminator : Terminator
  wires:
  In1/1 -> Terminator/1

== system lib_accessory2/SubLibraries/mechanical power logging/f ==
  In1 : Inport  Port=1  LatchInput=off
  Terminator : Terminator
  wires:
  In1/1 -> Terminator/1

== system lib_accessory2/SubLibraries/mechanical power logging/f1 ==
  In1 : Inport  Port=1  LatchInput=off
  Terminator : Terminator
  wires:
  In1/1 -> Terminator/1

== system lib_accessory2/SubLibraries/variable mechanical load --simulink implementation--/AC ==
  angular  speed of engine  shaft (rad/s) : Inport  Port=1  LatchInput=off
  elapsed time since start of simulation (s) : Inport  Port=2  LatchInput=off
  Look-Up Table (2-D) : simulink3/Functions & Tables/Look-Up Table (2-D)  x=map_spd  y=map_load  t=pwr_map
  Sat : Saturate  UpperLimit=1.0  LowerLimit=0.0  LinearizeAsGain=on
  Sat1 : Saturate  UpperLimit=maxSpd  LowerLimit=minSpd  LinearizeAsGain=on
  device duty  schedule by time : Subsystem  mask(Repeating table){t=acc_duty(:,1), y=acc_duty(:,2)}
      mask prompts: t "Input values:"; y "Output values:"
      mask help:
      | Repeating table.
      | Enter values of input and output for first cycle.
      mask init:
      | period = max(@1);
      settings: RTWFcnNameOpts=Auto  RTWFileNameOpts=Auto
      mask Help: Repeats cycle given in table. Input values should be monotonically increasing.
  powr required by device (W) : Outport  Port=1
  "duty cycle (1=\"on full power\" & 0=\"off\")" : Outport  Port=2
  wires:
  Sat1/1 -> Look-Up Table (2-D)/1
  angular  speed of engine  shaft (rad/s)/1 -> Sat1/1
  Sat/1 -> Look-Up Table (2-D)/2, "duty cycle (1=\"on full power\" & 0=\"off\")"/1
  device duty  schedule by time/1(out_1) -> Sat/1
  elapsed time since start of simulation (s)/1 -> device duty  schedule by time/1(distance travelled (m))
  Look-Up Table (2-D)/1 -> powr required by device (W)/1

== system lib_accessory2/SubLibraries/variable mechanical load --simulink implementation--/Air Compressor ==
  angular  speed of engine  shaft (rad/s) : Inport  Port=1  LatchInput=off
  elapsed time since start of simulation (s) : Inport  Port=2  LatchInput=off
  Look-Up Table (2-D) : simulink3/Functions & Tables/Look-Up Table (2-D)  x=map_spd  y=map_load  t=pwr_map
  Sat : Saturate  UpperLimit=1.0  LowerLimit=0.0  LinearizeAsGain=on
  Sat1 : Saturate  UpperLimit=maxSpd  LowerLimit=minSpd  LinearizeAsGain=on
  device duty  schedule by time : Subsystem  mask(Repeating table){t=acc_duty(:,1), y=acc_duty(:,2)}
      mask prompts: t "Input values:"; y "Output values:"
      mask help:
      | Repeating table.
      | Enter values of input and output for first cycle.
      mask init:
      | period = max(@1);
      settings: RTWFcnNameOpts=Auto  RTWFileNameOpts=Auto
      mask Help: Repeats cycle given in table. Input values should be monotonically increasing.
  powr required by device (W) : Outport  Port=1
  "duty cycle (1=\"on full power\" & 0=\"off\")" : Outport  Port=2
  wires:
  Sat1/1 -> Look-Up Table (2-D)/1
  angular  speed of engine  shaft (rad/s)/1 -> Sat1/1
  Sat/1 -> Look-Up Table (2-D)/2, "duty cycle (1=\"on full power\" & 0=\"off\")"/1
  device duty  schedule by time/1(out_1) -> Sat/1
  elapsed time since start of simulation (s)/1 -> device duty  schedule by time/1(distance travelled (m))
  Look-Up Table (2-D)/1 -> powr required by device (W)/1

== system lib_accessory2/SubLibraries/variable mechanical load --simulink implementation--/Alternator ==
  angular  speed of engine  shaft (rad/s) : Inport  Port=1  LatchInput=off
  load on device (W) : Inport  Port=2  LatchInput=off
  Constant : Constant  Value=0.0
  Constant1 : Constant  Value=eps
  Gain : Gain  Gain=1/conv_eff  Multiplication=Element-wise(K.*u)  SaturateOnIntegerOverflow=on
  Look-Up Table : Lookup  InputValues=map_spd  OutputValues=max_pwr
  Look-Up Table (2-D) : simulink3/Functions & Tables/Look-Up Table (2-D)  x=map_spd  y=map_load  t=pwr_map
  Product : Product  Inputs=*/  Multiplication=Element-wise(.*)  SaturateOnIntegerOverflow=on
  Relational Operator : RelationalOperator  Operator=~=
  Saturation : Saturate  UpperLimit=1.0  LowerLimit=0.0  LinearizeAsGain=on
  Saturation1 : Saturate  UpperLimit=maxSpd  LowerLimit=minSpd  LinearizeAsGain=on
  Switch : Switch  Threshold=0.5
  powr required by device (W) : Outport  Port=1
  wires:
  Switch/1 -> Product/2
  Constant1/1 -> Switch/3
  Relational Operator/1 -> Switch/2
  Constant/1 -> Relational Operator/2
  Look-Up Table/1 -> Switch/1, Relational Operator/1
  Saturation/1 -> Look-Up Table (2-D)/2
  Product/1 -> Saturation/1
  [spd] -> Look-Up Table/1
  Gain/1 -> Product/1
  Saturation1/1 -> [spd]
  [spd] -> Look-Up Table (2-D)/1
  angular  speed of engine  shaft (rad/s)/1 -> Saturation1/1
  Look-Up Table (2-D)/1 -> powr required by device (W)/1
  load on device (W)/1 -> Gain/1

== system lib_accessory2/SubLibraries/variable mechanical load --simulink implementation--/Power Steering ==
  angular  speed of engine  shaft (rad/s) : Inport  Port=1  LatchInput=off
  elapsed time since start of simulation (s) : Inport  Port=2  LatchInput=off
  Look-Up Table (2-D) : simulink3/Functions & Tables/Look-Up Table (2-D)  x=map_spd  y=map_load  t=pwr_map
  Sat : Saturate  UpperLimit=1.0  LowerLimit=0.0  LinearizeAsGain=on
  Sat1 : Saturate  UpperLimit=maxSpd  LowerLimit=minSpd  LinearizeAsGain=on
  device duty  schedule by time : Subsystem  mask(Repeating table){t=acc_duty(:,1), y=acc_duty(:,2)}
      mask prompts: t "Input values:"; y "Output values:"
      mask help:
      | Repeating table.
      | Enter values of input and output for first cycle.
      mask init:
      | period = max(@1);
      settings: RTWFcnNameOpts=Auto  RTWFileNameOpts=Auto
      mask Help: Repeats cycle given in table. Input values should be monotonically increasing.
  powr required by device (W) : Outport  Port=1
  "duty cycle (1=\"on full power\" & 0=\"off\")" : Outport  Port=2
  wires:
  Sat1/1 -> Look-Up Table (2-D)/1
  angular  speed of engine  shaft (rad/s)/1 -> Sat1/1
  Sat/1 -> Look-Up Table (2-D)/2, "duty cycle (1=\"on full power\" & 0=\"off\")"/1
  device duty  schedule by time/1(out_1) -> Sat/1
  elapsed time since start of simulation (s)/1 -> device duty  schedule by time/1(distance travelled (m))
  Look-Up Table (2-D)/1 -> powr required by device (W)/1
